simulink model "Full_system_1DOF_clock"  (R2015b)
settings: Solver=ode45  StartTime=0.0  StopTime=.7  MaxStep=1e-3  RelTol=1e-12
values from neighbouring files (symbols this model uses):
  a_hat = SC_xyz(2,:)/norm(SC_xyz(2,:))    [init_sim_1DOF.m]
  B_m = 0.5*8815e-4    (= 0.44075)    [init_sim_3DOF.m]
  c_B = 0    [init_sim_1DOF.m]    (also in init_sim_4DOF.m)
  OS_Inertia = 1e-9*[13894080.33 -19869.26 46055.05 ... (first row only)    [init_sim_1DOF.m]    (also in init_sim_3DOF.m; init_sim_4DOF.m; init_sim_6DOF.m = 1e-9*[15414004.18 -17587.97 46447.37)
  OS_init_omega = 0    [init_sim_1DOF.m]    (also in init_sim_3DOF.m; init_sim_4DOF.m = [0 0 0]'; init_sim_6DOF.m = [0 0 0]')
  OS_rotation = 0    [init_sim_1DOF.m]    (also in init_sim_3DOF.m; init_sim_4DOF.m = [0 0 0]'; init_sim_6DOF.m = [0 0 0]')
  T = .7    (= 0.7)    [init_sim_1DOF.m]
undefined symbols (not defined in the file or in its folder): EM_mu, EM_xyz, origin, OS_mu_0, OS_xyz_0
settings Model: Creator=user  LastModifiedBy=user
settings DataIOCC: SaveFormat=Array
settings DebuggingCC: SolverPrmCheckMsg=warning
settings HardwareCC: ProdBitPerPointer=32  ProdLargestAtomicFloat=None  ProdIntDivRoundTo=Undefined  ProdEndianess=Unspecified  ProdWordSize=32  ProdHWDeviceType=32-bit Generic
settings GRTTargetCC: GeneratePreprocessorConditionals=Disable all
settings ConfigComp: CovModelRefEnable=Off  CovSFcnEnable=off

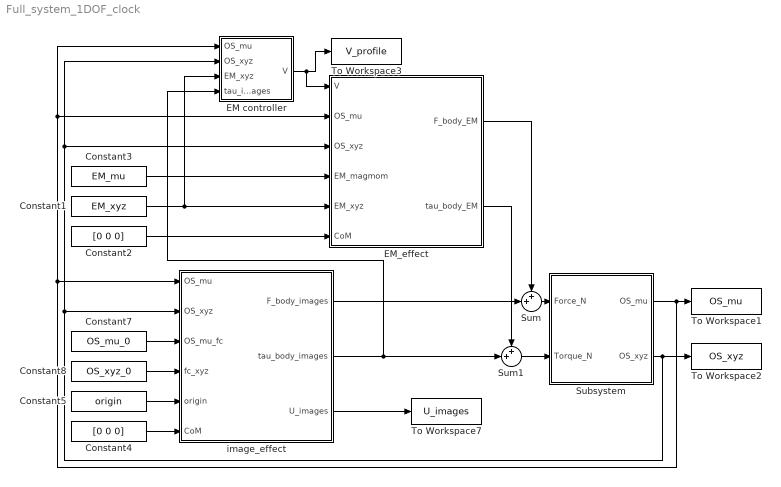
== system Full_system_1DOF_clock ==
  Constant1 : Constant  Value=EM_xyz
  Constant2 : Constant  Value=[0 0 0]
  Constant3 : Constant  Value=EM_mu
  Constant4 : Constant  Value=[0 0 0]
  Constant5 : Constant  Value=origin
  Constant7 : Constant  Value=OS_mu_0  VectorParams1D=off
  Constant8 : Constant  Value=OS_xyz_0
  EM controller : Subsystem
  EM_effect : MATLAB Function  TreatAsAtomicUnit=on
  Subsystem : Subsystem
  Sum : Sum  Inputs=++|
  Sum1 : Sum  Inputs=++|
  To Workspace1 : ToWorkspace  VariableName=OS_mu  SaveFormat=Timeseries  SampleTime=-1
      settings: Save2DSignal=2-D array (concatenate along first dimension)
  To Workspace2 : ToWorkspace  VariableName=OS_xyz  SaveFormat=Timeseries  SampleTime=-1
      settings: Save2DSignal=2-D array (concatenate along first dimension)
  To Workspace3 : ToWorkspace  VariableName=V_profile  SaveFormat=Timeseries  SampleTime=-1
      settings: Save2DSignal=2-D array (concatenate along first dimension)
  To Workspace7 : ToWorkspace  VariableName=U_images  SaveFormat=Timeseries  SampleTime=-1
      settings: Save2DSignal=2-D array (concatenate along first dimension)
  image_effect : MATLAB Function  TreatAsAtomicUnit=on
  wires:
  Constant3/1 -> EM_effect/4(EM_magmom)
  Constant1/1 -> EM_effect/5(EM_xyz), EM controller/3(EM_xyz)
  Constant2/1 -> EM_effect/6(CoM)
  Constant7/1 -> image_effect/3(OS_mu_fc)
  Constant8/1 -> image_effect/4(fc_xyz)
  Constant5/1 -> image_effect/5(origin)
  Constant4/1 -> image_effect/6(CoM)
  image_effect/3(U_images) -> To Workspace7/1
  Subsystem/1(OS_mu) -> EM_effect/2(OS_mu), EM controller/1(OS_mu), image_effect/1(OS_mu), To Workspace1/1
  Subsystem/2(OS_xyz) -> To Workspace2/1, EM_effect/3(OS_xyz), EM controller/2(OS_xyz), image_effect/2(OS_xyz)
  image_effect/1(F_body_images) -> Sum/2
  EM_effect/1(F_body_EM) -> Sum/1
  Sum/1 -> Subsystem/1(Force_N)
  EM_effect/2(tau_body_EM) -> Sum1/1
  Sum1/1 -> Subsystem/2(Torque_N)
  image_effect/2(tau_body_images) -> Sum1/2, EM controller/4(tau_images)
  EM controller/1(V) -> EM_effect/1(V), To Workspace3/1

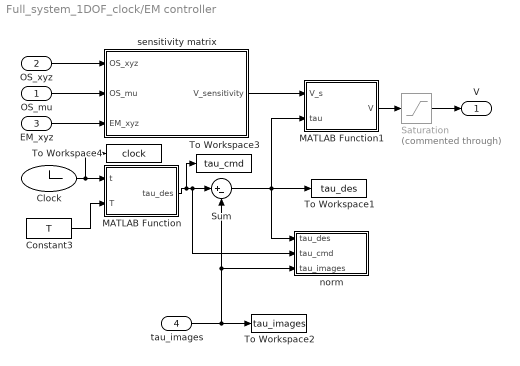
== system Full_system_1DOF_clock/EM controller ==
  OS_mu : Inport
  OS_xyz : Inport  Port=2
  EM_xyz : Inport  Port=3
  tau_images : Inport  Port=4
  Clock : Clock
  Constant3 : Constant  Value=T
  MATLAB Function : MATLAB Function  TreatAsAtomicUnit=on
  MATLAB Function1 : MATLAB Function  TreatAsAtomicUnit=on
  Saturation : Saturate  Commented=through  UpperLimit=12  LowerLimit=-12
  Sum : Sum  Inputs=|+-
  To Workspace1 : ToWorkspace  VariableName=tau_des  SaveFormat=Timeseries  SampleTime=-1
      settings: Save2DSignal=2-D array (concatenate along first dimension)
  To Workspace2 : ToWorkspace  VariableName=tau_images  SaveFormat=Timeseries  SampleTime=-1
      settings: Save2DSignal=2-D array (concatenate along first dimension)
  To Workspace3 : ToWorkspace  VariableName=tau_cmd  SaveFormat=Timeseries  SampleTime=-1
      settings: Save2DSignal=2-D array (concatenate along first dimension)
  To Workspace4 : ToWorkspace  VariableName=clock  SaveFormat=Timeseries  SampleTime=-1
      settings: Save2DSignal=2-D array (concatenate along first dimension)
  norm : Subsystem
  sensitivity matrix : MATLAB Function  TreatAsAtomicUnit=on
  V : Outport
  wires:
  OS_mu/1 -> sensitivity matrix/2(OS_mu)
  sensitivity matrix/1(V_sensitivity) -> MATLAB Function1/1(V_s)
  EM_xyz/1 -> sensitivity matrix/3(EM_xyz)
  OS_xyz/1 -> sensitivity matrix/1(OS_xyz)
  Sum/1 -> norm/1(tau_des), To Workspace1/1, MATLAB Function1/2(tau)
  MATLAB Function/1(tau_des) -> norm/2(tau_cmd), Sum/1, To Workspace3/1
  Clock/1 -> To Workspace4/1, MATLAB Function/1(t)
  tau_images/1 -> Sum/2, norm/3(tau_images), To Workspace2/1
  Constant3/1 -> MATLAB Function/2(T)
  MATLAB Function1/1(V) -> Saturation/1
  Saturation/1 -> V/1

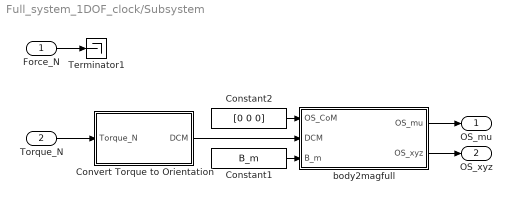
== system Full_system_1DOF_clock/Subsystem ==
  Force_N : Inport
  Torque_N : Inport  Port=2
  Constant1 : Constant  Value=B_m
  Constant2 : Constant  Value=[0 0 0]
  Convert Torque to Orientation : Subsystem
  Terminator1 : Terminator
  body2magfull : MATLAB Function  TreatAsAtomicUnit=on
  OS_mu : Outport
  OS_xyz : Outport  Port=2
  wires:
  body2magfull/2(OS_xyz) -> OS_xyz/1
  body2magfull/1(OS_mu) -> OS_mu/1
  Force_N/1 -> Terminator1/1
  Constant2/1 -> body2magfull/1(OS_CoM)
  Torque_N/1 -> Convert Torque to Orientation/1(Torque_N)
  Convert Torque to Orientation/1(DCM) -> body2magfull/2(DCM)
  Constant1/1 -> body2magfull/3(B_m)

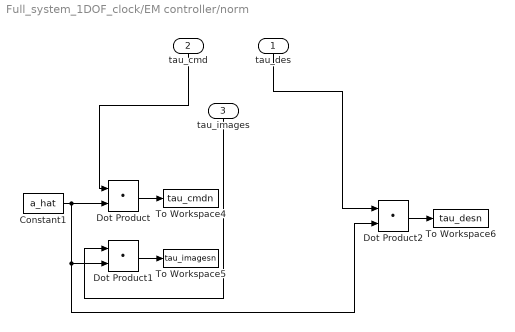
== system Full_system_1DOF_clock/EM controller/norm ==
  tau_des : Inport
  tau_cmd : Inport  Port=2
  tau_images : Inport  Port=3
  Constant1 : Constant  Value=a_hat
  Dot Product : DotProduct  InputSameDT=on  OutDataTypeStr=Inherit: Inherit via internal rule
  Dot Product1 : DotProduct  InputSameDT=on  OutDataTypeStr=Inherit: Inherit via internal rule
  Dot Product2 : DotProduct  InputSameDT=on  OutDataTypeStr=Inherit: Inherit via internal rule
  To Workspace4 : ToWorkspace  VariableName=tau_cmdn  SaveFormat=Timeseries  SampleTime=-1
      settings: Save2DSignal=2-D array (concatenate along first dimension)
  To Workspace5 : ToWorkspace  VariableName=tau_imagesn  SaveFormat=Timeseries  SampleTime=-1
      settings: Save2DSignal=2-D array (concatenate along first dimension)
  To Workspace6 : ToWorkspace  VariableName=tau_desn  SaveFormat=Timeseries  SampleTime=-1
      settings: Save2DSignal=2-D array (concatenate along first dimension)
  wires:
  tau_images/1 -> Dot Product1/1
  tau_cmd/1 -> Dot Product/1
  tau_des/1 -> Dot Product2/1
  Constant1/1 -> Dot Product2/2, Dot Product1/2, Dot Product/2
  Dot Product2/1 -> To Workspace6/1
  Dot Product/1 -> To Workspace4/1
  Dot Product1/1 -> To Workspace5/1

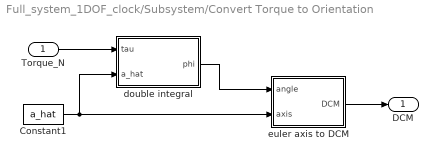
== system Full_system_1DOF_clock/Subsystem/Convert Torque to Orientation ==
  Torque_N : Inport
  Constant1 : Constant  Value=a_hat
  double integral : Subsystem
  euler axis to DCM : Subsystem
  DCM : Outport
  wires:
  Constant1/1 -> double integral/2(a_hat), euler axis to DCM/2(axis)
  euler axis to DCM/1(DCM) -> DCM/1
  Torque_N/1 -> double integral/1(tau)
  double integral/1(phi) -> euler axis to DCM/1(angle)

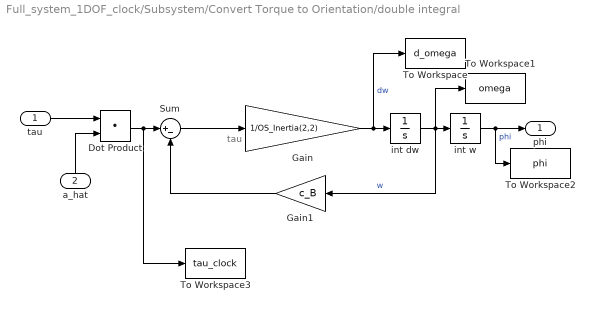
== system Full_system_1DOF_clock/Subsystem/Convert Torque to Orientation/double integral ==
  note: tau
  tau : Inport
  a_hat : Inport  Port=2
  Dot Product : DotProduct  InputSameDT=on  OutDataTypeStr=Inherit: Inherit via internal rule
  Gain : Gain  Gain=1/OS_Inertia(2,2)
  Gain1 : Gain  Gain=c_B
  Sum : Sum  Inputs=|+-
  To Workspace : ToWorkspace  VariableName=d_omega  SaveFormat=Timeseries  SampleTime=-1
  To Workspace1 : ToWorkspace  VariableName=omega  SaveFormat=Timeseries  SampleTime=-1
  To Workspace2 : ToWorkspace  VariableName=phi  SaveFormat=Timeseries  SampleTime=-1
  To Workspace3 : ToWorkspace  VariableName=tau_clock  SaveFormat=Timeseries  SampleTime=-1
  int dw : Integrator  InitialCondition=OS_init_omega
  int w : Integrator  InitialCondition=OS_rotation
  phi : Outport
  wires:
  a_hat/1 -> Dot Product/2
  Gain/1 -> To Workspace/1, int dw/1  "dw"
  int dw/1 -> Gain1/1, To Workspace1/1, int w/1  "w"
  int w/1 -> To Workspace2/1, phi/1  "phi"
  tau/1 -> Dot Product/1
  Sum/1 -> Gain/1
  Dot Product/1 -> To Workspace3/1, Sum/1
  Gain1/1 -> Sum/2

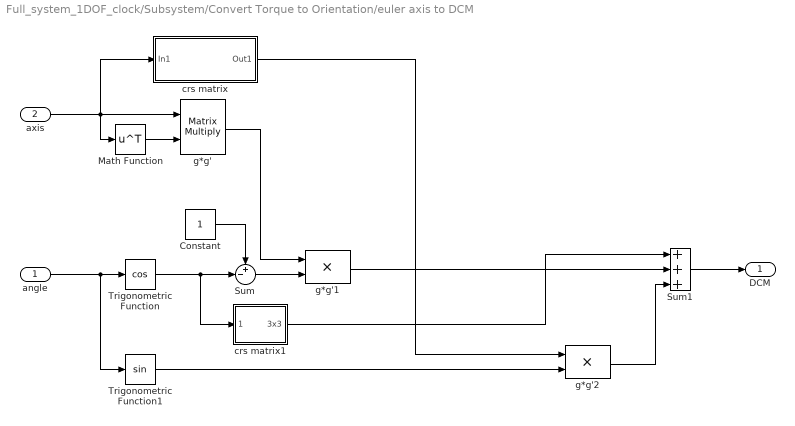
== system Full_system_1DOF_clock/Subsystem/Convert Torque to Orientation/euler axis to DCM ==
  angle : Inport
  axis : Inport  Port=2
  Constant : Constant
  Math Function : Math  Operator=transpose  SaturateOnIntegerOverflow=on
  Sum : Sum  Inputs=+-|  SaturateOnIntegerOverflow=on
  Sum1 : Sum  Inputs=+++  SaturateOnIntegerOverflow=on
  Trigonometric Function : Trigonometry  Operator=cos
  Trigonometric Function1 : Trigonometry
  crs matrix : Subsystem
  crs matrix1 : Subsystem
  g*g' : Product  Multiplication=Matrix(*)  SaturateOnIntegerOverflow=on  OutDataTypeStr=Inherit: Same as first input
  g*g'1 : Product  SaturateOnIntegerOverflow=on  OutDataTypeStr=Inherit: Same as first input
  g*g'2 : Product  SaturateOnIntegerOverflow=on  OutDataTypeStr=Inherit: Same as first input
  DCM : Outport
  wires:
  g*g'2/1 -> Sum1/3
  crs matrix1/1(3x3) -> Sum1/1
  Sum1/1 -> DCM/1
  crs matrix/1(Out1) -> g*g'2/1
  Trigonometric Function1/1 -> g*g'2/2
  g*g'1/1 -> Sum1/2
  g*g'/1 -> g*g'1/1
  Math Function/1 -> g*g'/2
  axis/1 -> crs matrix/1(In1), Math Function/1, g*g'/1
  Sum/1 -> g*g'1/2
  Constant/1 -> Sum/1
  Trigonometric Function/1 -> crs matrix1/1(make), Sum/2
  angle/1 -> Trigonometric Function1/1, Trigonometric Function/1

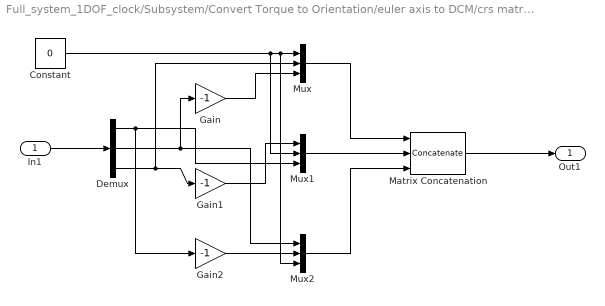
== system Full_system_1DOF_clock/Subsystem/Convert Torque to Orientation/euler axis to DCM/crs matrix ==
  In1 : Inport
  Constant : Constant  Value=0
  Demux : Demux  Outputs=3
  Gain : Gain  Gain=-1  SaturateOnIntegerOverflow=on  OutDataTypeStr=Inherit: Same as input  ParamDataTypeStr=Inherit: Same as input
  Gain1 : Gain  Gain=-1  SaturateOnIntegerOverflow=on  OutDataTypeStr=Inherit: Same as input  ParamDataTypeStr=Inherit: Same as input
  Gain2 : Gain  Gain=-1  SaturateOnIntegerOverflow=on  OutDataTypeStr=Inherit: Same as input  ParamDataTypeStr=Inherit: Same as input
  Matrix Concatenation : Concatenate  NumInputs=3  Mode=Multidimensional array  ConcatenateDimension=2
  Mux : Mux  Inputs=3
  Mux1 : Mux  Inputs=3
  Mux2 : Mux  Inputs=3
  Out1 : Outport
  wires:
  Matrix Concatenation/1 -> Out1/1
  Gain2/1 -> Mux2/2
  Mux2/1 -> Matrix Concatenation/3
  Mux1/1 -> Matrix Concatenation/2
  Demux/1 -> Gain2/1, Mux1/3
  Gain1/1 -> Mux1/1
  Mux/1 -> Matrix Concatenation/1
  Gain/1 -> Mux/3
  Demux/2 -> Mux2/1, Gain/1
  Demux/3 -> Gain1/1, Mux/2
  Constant/1 -> Mux2/3, Mux/1, Mux1/2
  In1/1 -> Demux/1

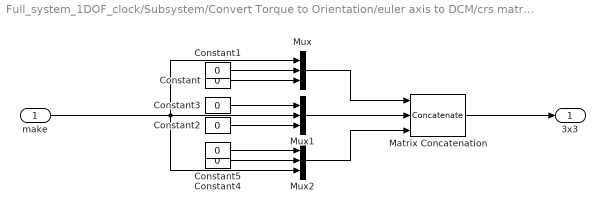
== system Full_system_1DOF_clock/Subsystem/Convert Torque to Orientation/euler axis to DCM/crs matrix1 ==
  make : Inport
  Constant{,1..5} (6 alike) : Constant  Value=0
  Matrix Concatenation : Concatenate  NumInputs=3  Mode=Multidimensional array  ConcatenateDimension=2
  Mux : Mux  Inputs=3
  Mux1 : Mux  Inputs=3
  Mux2 : Mux  Inputs=3
  3x3 : Outport
  wires:
  Constant5/1 -> Mux2/1
  Constant4/1 -> Mux2/2
  Constant3/1 -> Mux1/1
  Constant2/1 -> Mux1/3
  Constant1/1 -> Mux/2
  Constant/1 -> Mux/3
  Matrix Concatenation/1 -> 3x3/1
  Mux2/1 -> Matrix Concatenation/3
  Mux1/1 -> Matrix Concatenation/2
  Mux/1 -> Matrix Concatenation/1
  make/1 -> Mux2/3, Mux1/2, Mux/1

== matlab function Full_system_1DOF_clock/EM controller/MATLAB Function ==
  data: t input; tau_des output; T input
function tau_des = slew(t,T)
%#codegen
%direction cosine matrix to rotate one trio to the next about
%superconductor 1
phi=72*pi/180;
SC_xyz=[0,0.0622991367861173,0.100802120789717;-0.0622991367861173,0.100802120789717,0;0.0622991367861173,0.100802120789717,0];
a=SC_xyz(2,:)/norm(SC_xyz(2,:)); %the euler axis, superconductor 1 in this case
%to perform a slew, phi will change over time. in this case a versine
% T=.7; %time to complete maneuver
phi_ddt=0.5*phi*(pi/T)^2*cos(pi*t/T); %angular acceleration about axis over time

%angular acceleration may be representation by [magnitude of angular
%acceleration] * unit vector of direction of angular acceleration
%in our case, phi_ddt*a
alpha=a'*phi_ddt; %each column is an acceleration needed at each time step

OS_Inertia=[0.0138940803300000,-1.98692600000000e-05,4.60550500000000e-05;-1.98692600000000e-05,0.0128627100800000,1.65018000000000e-05;4.60550500000000e-05,1.65018000000000e-05,0.0138967280000000];
%each column is the body torque needed to accomplish the versine slew
tau_des=OS_Inertia(2,2)*alpha;

== matlab function Full_system_1DOF_clock/EM controller/MATLAB Function1 ==
  data: V_s input; tau input; V output
function V = driver(V_s,tau)
%#codegen
V=pinv(V_s(4:6,:))*tau;

== matlab function Full_system_1DOF_clock/Subsystem/body2magfull ==
  data: OS_CoM input; OS_mu output; DCM input; OS_xyz output; B_m input
function [OS_mu,OS_xyz] = body2mag(OS_CoM,DCM,B_m)
%#codegen
tau=(1+sqrt(5))/2;
OS_xyz=[0 1 tau;
    -1 tau 0;
    1 tau 0;
    0 1 -tau;
    0 -1 tau;
    0 -1 -tau;
    1 -tau 0;
    -1 -tau 0;
    tau 0 1;
    tau 0 -1;
    -tau 0 -1;
    -tau 0 1];
%^the coordinate points of an icosahedron
D=20.3/100; %m the diameter of the OS
magd=1.905/100; %m the diameter of the 0.75 inch spherical magnets to use
rM=(D-magd)/2; %m this radius corresponds to the center of the magnets 
%so that the magnets are flush against the OS surface
OS_magmom=zeros(size(OS_xyz));
for i=1:size(OS_xyz,1)
    OS_magmom(i,:)=(DCM*OS_xyz(i,:)'/norm(OS_xyz(i,:)))';
    OS_xyz(i,:)=OS_magmom(i,:)*rM+OS_CoM';
end
%the permeability of free space, mu_0
mu_0=4*pi*10^-7; %N/A^2

%distance from the center of the magnet to its surface
d_m=1.905/2/100; %m

%the estimated magnetic dipole moment magnitude for each magnet on the OS
%surface
OS_mu=2*pi*B_m*d_m^3/mu_0*OS_magmom;

== matlab function Full_system_1DOF_clock/EM controller/sensitivity matrix ==
  data: OS_xyz input; V_sensitivity output; OS_mu input; EM_xyz input
function V_sensitivity=calculate_voltage(OS_xyz, OS_mu, EM_xyz)
%% Calculate the needed electromagnet voltage with a pseudoinverse
    %initialize a placeholder for the pseudoinverse
    V_sensitivity=zeros(6,6);
    
    %sift through all the electromagnets to back out portion of force
    %and torque generated from each individually
    for i=1:6 
        %initialize sum of electromagnet contribution acting on each
        %permanent magnet due to electromagnet i
        dF_tot=zeros(1,3); 
        dtau_tot=zeros(1,3);
        %calculate electromagnet affect on force and torque on body through
        %all the permanent magnets
        for j=1:size(OS_xyz,2) 
            %in this case, the magnetic moment dipole being acted on is the 
            %permanent magnet, following Villani convention
            mu_mag_i=OS_mu(j,:);
            pos_mag_i=OS_xyz(j,:);
            %the magnetic moment dipole acting on magnet i is the
            %electromagnet
            pos_mag_j=EM_xyz(i,:);
            mu_mag_j=-EM_xyz(i,:)/norm(EM_xyz(i,:));
            %calculate_dV is a variation of villani. Villani requires mu
            %components and the position vector between them. Within
            %calculate_dV, the electromagnet's magnetic dipole/voltage is
            %substituted for force and torque per unit Volt
            [dF_dV,dtau_dV]=calculate_dV(mu_mag_i,pos_mag_i,mu_mag_j,pos_mag_j);
            %sum over each permanent magnet
            dF_tot=dF_tot+dF_dV;
            dtau_tot=dtau_tot+dtau_dV+cross(dF_tot,pos_mag_i);
        end
        %fill in the portion of the pseudoinverse needed to calculate
        %electromagnetic contribution
        V_sensitivity(:,i)=[dF_tot';dtau_tot'];
    end
end

== matlab function Full_system_1DOF_clock/EM_effect ==
  data: V input; OS_mu input; F_body_EM output; OS_xyz input; EM_magmom input; EM_xyz input; tau_body_EM output; CoM input
function [F_body_EM,tau_body_EM]=EM_effect(V,OS_mu,OS_xyz,EM_magmom,EM_xyz,CoM)
%% Calculate the needed electromagnet voltage with a pseudoinverse
    %initialize a placeholder for the pseudoinverse
    A=zeros(6,length(V));
    
    %sift through all the electromagnets to back out portion of force
    %and torque generated from each individually
    for i=1:length(V) 
        %initialize sum of electromagnet contribution acting on each
        %permanent magnet due to electromagnet i
        dF_tot=zeros(1,3); 
        dtau_tot=zeros(1,3);
        %calculate electromagnet affect on force and torque on body through
        %all the permanent magnets
        for j=1:size(OS_xyz,1) 
            %in this case, the magnetic moment dipole being acted on is the 
            %permanent magnet, following Villani convention
            mu_mag_i=OS_mu(j,:);
            pos_mag_i=OS_xyz(j,:);
            %the magnetic moment dipole acting on magnet i is the
            %electromagnet
            mu_mag_j=EM_magmom(i,:);
            pos_mag_j=EM_xyz(i,:);
            %calculate_dV is a variation of villani. Villani requires mu
            %components and the position vector between them. Within
            %calculate_dV, the electromagnet's magnetic dipole/voltage is
            %substituted for force and torque per unit Volt
            [dF_dV,dtau_dV]=calculate_dV(mu_mag_i,pos_mag_i,mu_mag_j,pos_mag_j);
            %sum over each permanent magnet
            dF_tot=dF_tot+dF_dV;
            dtau_tot=dtau_tot+dtau_dV+cross(dF_tot,pos_mag_i-CoM');
        end
        %fill in the portion of the pseudoinverse needed to calculate
        %electromagnetic contribution
        A(:,i)=[dF_tot';dtau_tot'];
    end
    %voltage calculated for this time step using the pseudoinverse
    y=A*V;
    F_body_EM=y(1:3);
    tau_body_EM=y(4:6);
end
    
function [dF_dV,dtau_dV]=calculate_dV(mu_mag_i,pos_mag_i,mu_mag_j,pos_mag_j)
%this function calculates force and torque per voltage acting on the 
%source magnet from an electromagnet
%mu_mag_i is the magnetic moment dipole of a magnet i
%mu_mag_j is the magnetic moment dipole of the electromagnet
%pos_mag_i is the position of the magnet i
%pos_mag_j is the position of the electromagnet

%the following parameters follow Laura's past experiments
%area enclosed by the electromagnet's current loop
A=0.001829214; %m^2
%number of turns in the electromagnet
T=1060;
%resistance of electromagnet
R=16.8; %Ohmsa
%the permeability of free space, mu_0
mu_0=4*pi*10^-7; %N/A^2

%the following parameters are required by Villani's analytical equations
%for forces and torques on two magnetic dipoles
rho_mji=pos_mag_j-pos_mag_i;
mu_mj_dV=A*T/R*mu_mag_j;
%the voltage is directly proportional to the force and torque applied on
%the magnetic dipole, making the calculation linear and relatively easy

[dF_dV,dtau_dV]=villani(mu_0,mu_mj_dV,mu_mag_i,rho_mji);
%the dF_dV dtau_dV will be evaluated for each electromagnet
%where [F; tau]=[dF_dV;dtau_dV]*[V] 
%V is a 6x1 column vector consisting of V_n for electromagnet n
%F is a 3x1 column vector consisting of forces in the x, y, and z
%tau is a 3x1 column vector consisting of torques in the x, y, and z
%[dF_dV;dtau_dV] is a 6x6 matrix consisting of the contribution of force
%and torque per volt from each electromagnet

end

== matlab function Full_system_1DOF_clock/image_effect ==
  data: OS_mu input; F_body_images output; OS_xyz input; OS_mu_fc input; fc_xyz input; origin input; tau_body_images output; CoM input; U_images output
function [F_body_images,tau_body_images,U_images]=image_effect(OS_mu,OS_xyz,...
    OS_mu_fc,fc_xyz,origin,CoM)
%#codegen

%F_body_images is the total force on the body due to mobile and frozen
% image effects
%tau_body_images is the total torque on the body due to mobile and frozen
% image effects
%frozen_lists and mobile_lists keeps track of the individual mobile and
% frozen image effects
%OS_mu are the magnetic moment dipoles of the permanent magnets on the OS
%OS_xyz are the magnet positions on the OS
%OS_mu_fc are the field cooled magnetic moment dipoles of the permanent
% magnets on the OS
%fc_xyz are the field cooled positions of the permanent magnets on the OS
%origin is an arbitrary point on the superconductor surface that I have
% chosen to be the center of the superconductor disk surface

%F_body_sum and tau_body_sum is to keep track of the communative effort of
%all frozen and mobile images on magnet i, correlating to row i
F_body_sum=zeros(size(OS_mu,1),3);
tau_body_sum=zeros(size(OS_mu,1),3);
U_fsum=zeros(size(OS_mu,1),1);
U_msum=zeros(size(OS_mu,1),1);
%frozen_lists and mobile_lists goes more in depth than F_body_sum and
%tau_body_sum, storing the individual effect of every frozen and mobile
%image where:
%the first column represents magnet i
%the second column represents magnet j
%third to fifth columns represent force on magnet i due to j's image
%sixth to eighth columns represent torque on magnet i due to j's image
% frozen_lists=zeros(size(OS_mu,1)^2,8,size(origin,1));
% mobile_lists=zeros(size(OS_mu,1)^2,8,size(origin,1));


%% Sum frozen and mobile images across different superconductors and all magnets
for k=1:size(origin,1) %sift through all the superconductors
    %initialize row counter
    row=1;
    for i=1:size(OS_xyz,1) %sift through all the magnets i
        
        mu_mag_i=OS_mu(i,:);
        pos_mag_i=OS_xyz(i,:);
        O=origin(k,:);
        
        for j=1:size(OS_xyz,1) %sift through all the magnets j that generate images
            
            mu_mag_j=OS_mu(j,:);
            pos_mag_j=OS_xyz(j,:);
            mu_mag_fc=OS_mu_fc(j,:);
            pos_fc=fc_xyz(j,:);

            %find the contribution of each field cooled image on all the
            %permanent magnets
            effect='frozen';
            [F,tau,U]=calculate_Ftau(mu_mag_i,mu_mag_j,mu_mag_fc,...
                pos_mag_i,pos_mag_j,pos_fc,O,effect);

            F_body_sum(i,:)=F_body_sum(i,:)+F;
            tau_body_sum(i,:)=tau_body_sum(i,:)+tau+cross(pos_mag_i-CoM',F);
            U_fsum(i)=U_fsum(i)+U;
            %this list is for debugging storing all frozen image effects,
            %first column the magnet, second column the frozen image, 3:5
            %column the force, 6:8 the torque
%             frozen_lists(row,1,k)=i;
%             frozen_lists(row,2,k)=j;
%             frozen_lists(row,3:5,k)=F;
%             frozen_lists(row,6:8,k)=tau;      

            %find the contribution of this magnet's mobile image on
            %the i_th source magnet
            effect='mobile';
            [F,tau,U]=calculate_Ftau(mu_mag_i,mu_mag_j,mu_mag_fc,...
                pos_mag_i,pos_mag_j,pos_fc,O,effect);
            
            F_body_sum(i,:)=F_body_sum(i,:)+F;
            tau_body_sum(i,:)=tau_body_sum(i,:)+tau+cross(pos_mag_i-CoM',F);
            U_msum(i)=U_msum(i)+U;
            %this list is for debugging storing all mobile image effects,
            %first column the magnet, second column the frozen image, 3:5
            %column the force, 6:8 the torque
%             mobile_lists(row,1,k)=i;
%             mobile_lists(row,2,k)=j;
%             mobile_lists(row,3:5,k)=F;
%             mobile_lists(row,6:8,k)=tau;

            row=row+1;
        end
    end
end

%sum columns to get the total force and torque on the body
F_body_images=sum(F_body_sum,1)';
tau_body_images=sum(tau_body_sum,1)';
U_images=[sum(U_fsum) sum(U_msum)];
